simulink subsystem "battlimcheck"  (R2022b)
settings: Solver=VariableStepAuto  StartTime=0.0  StopTime=10.0  RelTol=1e-3
libraries: simulink x3
settings Model: Creator=serga  LastModifiedBy=serga

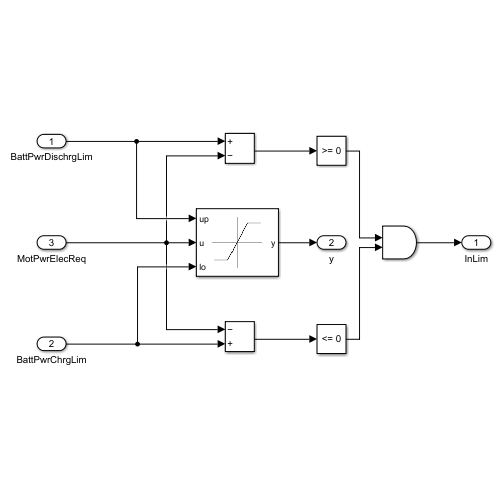
[thumbnail: Simulink's stored preview of the top-level diagram]
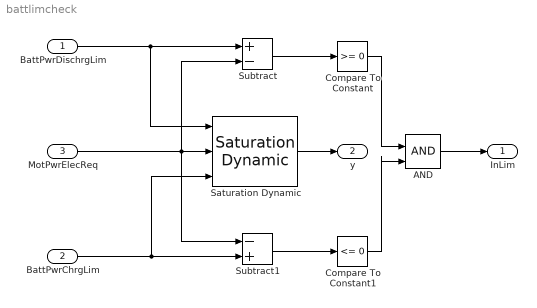
== system battlimcheck ==
  BattPwrDischrgLim : Inport
  BattPwrChrgLim : Inport  Port=2
  MotPwrElecReq : Inport  Port=3
  AND : Logic  IconShape=distinctive  AllPortsSameDT=off  OutDataTypeStr=boolean
  Compare To Constant : simulink/Logic and Bit Operations/Compare To Constant  relop=>=  const=0  OutDataTypeStr=boolean
  Compare To Constant1 : simulink/Logic and Bit Operations/Compare To Constant  relop=<=  const=0  OutDataTypeStr=boolean
  Saturation Dynamic : simulink/Discontinuities/Saturation Dynamic  OutMin=[]  OutMax=[]  OutDataTypeStr=Inherit: Same as second input  OutDataType=fixdt(1, 16)  OutScaling=2^-10  DoSatur=off
  Subtract : Sum  Inputs=+-
  Subtract1 : Sum  Inputs=-+
  InLim : Outport
  y : Outport  Port=2
  wires:
  BattPwrDischrgLim/1 -> Saturation Dynamic/1, Subtract/1
  MotPwrElecReq/1 -> Subtract/2, Subtract1/1, Saturation Dynamic/2
  BattPwrChrgLim/1 -> Saturation Dynamic/3, Subtract1/2
  Subtract/1 -> Compare To Constant/1
  Subtract1/1 -> Compare To Constant1/1
  Compare To Constant/1 -> AND/1
  Compare To Constant1/1 -> AND/2
  AND/1 -> InLim/1
  Saturation Dynamic/1 -> y/1
